simulink model "DIODE_2"  (Simulink 7.7)
settings: Solver=ode15s  StartTime=0.0  StopTime=0.2  MaxStep=0.001  RelTol=1e-3
libraries: fl_lib x18, elec_lib x14, nesl_utility x1
settings Model: Creator=Korisnik  LastModifiedBy=Korisnik

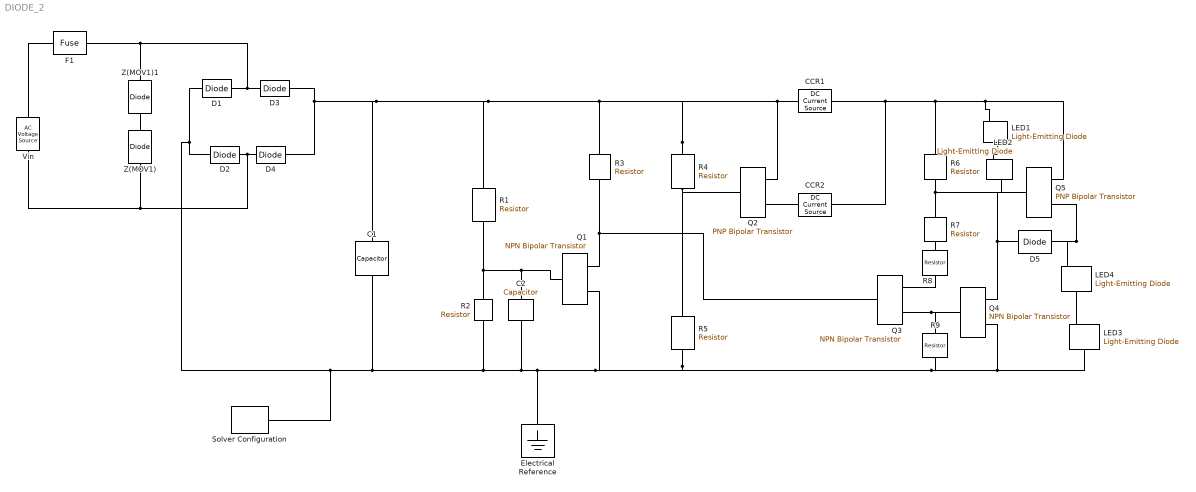
== system DIODE_2 ==
  C1 : fl_lib/Electrical/Electrical Elements/Capacitor  SystemSampleTime=-1  c=2.2 nF  v0=0 V  r=1e-6 Ohm  g=0 1/Ohm  i_Log=off  v_Log=off  vc_Log=off  LocalVarNames=|i|v|vc  LocalVarDescs=|i|v|Internal variable for voltage across capacitor term  LocalVarLogging=[0 0 0]
  C2 : fl_lib/Electrical/Electrical Elements/Capacitor  SystemSampleTime=-1  c=1 nF  v0=0 V  r=1e-6 Ohm  g=0 1/Ohm  i_Log=off  v_Log=off  vc_Log=off  LocalVarNames=|i|v|vc  LocalVarDescs=|i|v|Internal variable for voltage across capacitor term  LocalVarLogging=[0 0 0]
  CCR1 : elec_lib/Additional Components/SPICE-Compatible Components/Sources/DC Current Source  SystemSampleTime=-1  DC=50 mA  current_Log=off  voltage_Log=off  power_Log=off  LocalVarNames=|current|voltage|power  LocalVarDescs=|Current (A)|Voltage (V)|Power (W)  LocalVarLogging=[0 0 0]
  CCR2 : elec_lib/Additional Components/SPICE-Compatible Components/Sources/DC Current Source  SystemSampleTime=-1  DC=30 mA  current_Log=off  voltage_Log=off  power_Log=off  LocalVarNames=|current|voltage|power  LocalVarDescs=|Current (A)|Voltage (V)|Power (W)  LocalVarLogging=[0 0 0]
  D{1..4} (4 alike) : fl_lib/Electrical/Electrical Elements/Diode  SystemSampleTime=-1  Vf=0.68 V  Ron=0.3 Ohm  Goff=1e-8 1/Ohm  i_Log=off  v_Log=off  LocalVarNames=|i|v  LocalVarDescs=|i|v  LocalVarLogging=[0 0]
  D5 : fl_lib/Electrical/Electrical Elements/Diode  SystemSampleTime=-1  Vf=0.6 V  Ron=0.3 Ohm  Goff=1e-8 1/Ohm  i_Log=off  v_Log=off  LocalVarNames=|i|v  LocalVarDescs=|i|v  LocalVarLogging=[0 0]
  Electrical Reference : fl_lib/Electrical/Electrical Elements/Electrical Reference  SystemSampleTime=-1  i_Log=off  LocalVarNames=|i  LocalVarDescs=|i  LocalVarLogging=0
  F1 : elec_lib/Passive Devices/Fuse  SystemSampleTime=-1  I_rated=1 A  T_fuse=0 s  R_closed=0.01 Ohm  G_open=1e-8 1/Ohm  current_Log=off  voltage_Log=off  power_Log=off  LocalVarNames=|current|voltage|power  LocalVarDescs=|Current (A)|Voltage (V)|Power (W)  LocalVarLogging=[0 0 0]
  LED{1..4} (4 alike) : elec_lib/Sensors/Light-Emitting Diode  SystemSampleTime=-1  Gain=0.005 W/A  prmExp=1  I12=[ 0.0017 0.003 ] A  V12=[ 0.9 1.05 ] V  RS=0.1 Ohm  IS=5e-5 A  Tmeas=25 C  ec=10  C_param=1  CJ0=20 pF  VJ=1 V  Mgrad=0.5  Vvec=[ 0.1 10 100 ] V  Cvec=[ 15 10 2 ] pF  FC=0.5  T_param=1  IS_T2=1.8e-4 A  I1_T2=0.0034 A  V1_T2=1.05 V  Tmeas2=125 C  EG_param=1  EG=1.11 eV  XTI_param=1  XTI=3  Tdevice=25 C  LocalVarLogging=[]
  Q1 : elec_lib/Semiconductor Devices/NPN Bipolar Transistor  SystemSampleTime=-1  parameterization=1  prmDatasheet=1  prmEquCoeff=1  BF=100  IS=1e-14 A  VAF=200 V  hfe=100  hoe=5e-5 1/Ohm  Ic_h=1 mA  Vce_h=5 V  V1=0.55 V  I1=0.5 mA  BR=1  Tmeas=25 C  RC=0.01 Ohm  RE=1e-4 Ohm  RB=1 Ohm  C_BC=5 pF  C_BE=5 pF  TF=0 us  TR=0 us  hfe_T2=125  XTB=0  V1_T2=0.45 V  I1_T2=0.5 mA  Tmeas2=125 C  EG=1.11 eV  XTI=3  TdeviceDatasheet=25 C  TdeviceEquCoeff=25 C  LocalVarLogging=[]
  Q2 : elec_lib/Semiconductor Devices/PNP Bipolar Transistor  SystemSampleTime=-1  parameterization=1  prmDatasheet=1  prmEquCoeff=1  BF=100  IS=1e-14 A  VAF=200 V  hfe=100  hoe=5e-5 1/Ohm  Ic_h=-1 mA  Vce_h=-5 V  V1=-0.55 V  I1=-0.5 mA  BR=1  Tmeas=25 C  RC=0.01 Ohm  RE=1e-4 Ohm  RB=1 Ohm  C_BC=5 pF  C_BE=5 pF  TF=0 us  TR=0 us  hfe_T2=125  XTB=0  V1_T2=-0.45 V  I1_T2=-0.5 mA  Tmeas2=125 C  EG=1.11 eV  XTI=3  TdeviceDatasheet=25 C  TdeviceEquCoeff=25 C  LocalVarLogging=[]
  Q3 : elec_lib/Semiconductor Devices/NPN Bipolar Transistor  SystemSampleTime=-1  parameterization=1  prmDatasheet=1  prmEquCoeff=1  BF=100  IS=1e-14 A  VAF=200 V  hfe=100  hoe=5e-5 1/Ohm  Ic_h=1 mA  Vce_h=5 V  V1=0.55 V  I1=0.5 mA  BR=1  Tmeas=25 C  RC=0.01 Ohm  RE=1e-4 Ohm  RB=1 Ohm  C_BC=5 pF  C_BE=5 pF  TF=0 us  TR=0 us  hfe_T2=125  XTB=0  V1_T2=0.45 V  I1_T2=0.5 mA  Tmeas2=125 C  EG=1.11 eV  XTI=3  TdeviceDatasheet=25 C  TdeviceEquCoeff=25 C  LocalVarLogging=[]
  Q4 : elec_lib/Semiconductor Devices/NPN Bipolar Transistor  SystemSampleTime=-1  parameterization=1  prmDatasheet=1  prmEquCoeff=1  BF=100  IS=1e-14 A  VAF=200 V  hfe=100  hoe=5e-5 1/Ohm  Ic_h=1 mA  Vce_h=5 V  V1=0.55 V  I1=0.5 mA  BR=1  Tmeas=25 C  RC=0.01 Ohm  RE=1e-4 Ohm  RB=1 Ohm  C_BC=5 pF  C_BE=5 pF  TF=0 us  TR=0 us  hfe_T2=125  XTB=0  V1_T2=0.45 V  I1_T2=0.5 mA  Tmeas2=125 C  EG=1.11 eV  XTI=3  TdeviceDatasheet=25 C  TdeviceEquCoeff=25 C  LocalVarLogging=[]
  Q5 : elec_lib/Semiconductor Devices/PNP Bipolar Transistor  SystemSampleTime=-1  parameterization=1  prmDatasheet=1  prmEquCoeff=1  BF=100  IS=1e-14 A  VAF=200 V  hfe=100  hoe=5e-5 1/Ohm  Ic_h=-1 mA  Vce_h=-5 V  V1=-0.55 V  I1=-0.5 mA  BR=1  Tmeas=25 C  RC=0.01 Ohm  RE=1e-4 Ohm  RB=1 Ohm  C_BC=5 pF  C_BE=5 pF  TF=0 us  TR=0 us  hfe_T2=125  XTB=0  V1_T2=-0.45 V  I1_T2=-0.5 mA  Tmeas2=125 C  EG=1.11 eV  XTI=3  TdeviceDatasheet=25 C  TdeviceEquCoeff=25 C  LocalVarLogging=[]
  R1 : fl_lib/Electrical/Electrical Elements/Resistor  SystemSampleTime=-1  R=1 MOhm  i_Log=off  v_Log=off  LocalVarNames=|i|v  LocalVarDescs=|i|v  LocalVarLogging=[0 0]
  R2 : fl_lib/Electrical/Electrical Elements/Resistor  SystemSampleTime=-1  R=5.6 kOhm  i_Log=off  v_Log=off  LocalVarNames=|i|v  LocalVarDescs=|i|v  LocalVarLogging=[0 0]
  R3 : fl_lib/Electrical/Electrical Elements/Resistor  SystemSampleTime=-1  R=301 kOhm  i_Log=off  v_Log=off  LocalVarNames=|i|v  LocalVarDescs=|i|v  LocalVarLogging=[0 0]
  R4 : fl_lib/Electrical/Electrical Elements/Resistor  SystemSampleTime=-1  R=590 Ohm  i_Log=off  v_Log=off  LocalVarNames=|i|v  LocalVarDescs=|i|v  LocalVarLogging=[0 0]
  R5 : fl_lib/Electrical/Electrical Elements/Resistor  SystemSampleTime=-1  R=100 kOhm  i_Log=off  v_Log=off  LocalVarNames=|i|v  LocalVarDescs=|i|v  LocalVarLogging=[0 0]
  R6 : fl_lib/Electrical/Electrical Elements/Resistor  SystemSampleTime=-1  R=2.2 kOhm  i_Log=off  v_Log=off  LocalVarNames=|i|v  LocalVarDescs=|i|v  LocalVarLogging=[0 0]
  R7 : fl_lib/Electrical/Electrical Elements/Resistor  SystemSampleTime=-1  R=27 kOhm  i_Log=off  v_Log=off  LocalVarNames=|i|v  LocalVarDescs=|i|v  LocalVarLogging=[0 0]
  R8 : fl_lib/Electrical/Electrical Elements/Resistor  SystemSampleTime=-1  R=27 kOhm  i_Log=off  v_Log=off  LocalVarNames=|i|v  LocalVarDescs=|i|v  LocalVarLogging=[0 0]
  R9 : fl_lib/Electrical/Electrical Elements/Resistor  SystemSampleTime=-1  R=2.2 kOhm  i_Log=off  v_Log=off  LocalVarNames=|i|v  LocalVarDescs=|i|v  LocalVarLogging=[0 0]
  Solver Configuration : nesl_utility/Solver Configuration  SystemSampleTime=-1  PhysicalDomain=network_engine_domain  LeftPortType=input  RightPortType=generic  SubClassName=solver  Accelerate=off  Profile=off  ResidualTolerance=1e-9  MaxNonlinIter=3  MaxModeIter=2  DoFixedCost=off  UseLocalSampling=off  DoDC=off  LinearAlgebra=Sparse  LocalSolverSampleTime=.001  LocalSolverChoice=NE_BACKWARD_EULER_ADVANCER  UseLocalSolver=off
  Vin : fl_lib/Electrical/Electrical Sources/AC Voltage Source  SystemSampleTime=-1  amp=169.71 V  shift=0 rad  omega=60 Hz  i_Log=off  v_Log=off  LocalVarNames=|i|v  LocalVarDescs=|i|v  LocalVarLogging=[0 0]
  Z(MOV1) : elec_lib/Semiconductor Devices/Diode  SystemSampleTime=-1  ModelType=2  Vf=0.6 V  Ron=0.3 Ohm  Goff=1e-8 S  Rz=0.3 Ohm  Vz=150 V  C_PWL=5 pF  prmExp=1  I12=[ 0.0137 0.545 ] A  V12=[ 0.6 0.7 ] V  I1=0.0137 A  V1=0.6 V  RS=0.01 Ohm  IS=1e-12 A  Tmeas=25 C  ec=1  BV=Inf V  C_param=1  CJ0=5 pF  VJ=1 V  Mgrad=0.5  Vvec=[ 0.1 10 100 ] V  Cvec=[ 3.5 1 0.4 ] pF  FC=0.5  T_param=1  IS_T2=1.25e-7 A  I1_T2=0.245 A  V1_T2=0.5 V  Tmeas2=125 C  EG_param=1  EG=1.11 eV  XTI_param=1  XTI=3  dBVdT=0 V/K  Tdevice=25 C  LocalVarLogging=[]
  Z(MOV1)1 : elec_lib/Semiconductor Devices/Diode  SystemSampleTime=-1  ModelType=2  Vf=0.6 V  Ron=0.3 Ohm  Goff=1e-8 S  Rz=0.3 Ohm  Vz=150 V  C_PWL=5 pF  prmExp=1  I12=[ 0.0137 0.545 ] A  V12=[ 0.6 0.7 ] V  I1=0.0137 A  V1=0.6 V  RS=0.01 Ohm  IS=1e-12 A  Tmeas=25 C  ec=1  BV=Inf V  C_param=1  CJ0=5 pF  VJ=1 V  Mgrad=0.5  Vvec=[ 0.1 10 100 ] V  Cvec=[ 3.5 1 0.4 ] pF  FC=0.5  T_param=1  IS_T2=1.25e-7 A  I1_T2=0.245 A  V1_T2=0.5 V  Tmeas2=125 C  EG_param=1  EG=1.11 eV  XTI_param=1  XTI=3  dBVdT=0 V/K  Tdevice=25 C  LocalVarLogging=[]
  connections:
  Vin/RConn1 -- D2/RConn1 -- D4/LConn1 -- Z(MOV1)/LConn1
  F1/LConn1 -- Vin/LConn1
  R9/RConn1 -- Q4/RConn2 -- LED3/RConn1 -- R5/RConn1 -- Q1/RConn2 -- C2/RConn1 -- R2/RConn1 -- C1/RConn1 -- D1/LConn1 -- D2/LConn1 -- Solver Configuration/RConn1 -- Electrical Reference/LConn1
  R3/RConn1 -- Q1/RConn1 -- Q3/LConn1
  R4/RConn1 -- R5/LConn1 -- Q2/LConn1
  CCR2/LConn1 -- Q2/RConn2
  LED1/LConn2 -- R6/LConn1 -- CCR1/RConn1 -- CCR2/RConn1 -- Q5/RConn1
  R6/RConn1 -- R7/LConn1 -- Q5/LConn1
  R7/RConn1 -- R8/LConn1
  R9/LConn1 -- Q3/RConn2 -- Q4/LConn1
  R1/RConn1 -- R2/LConn1 -- C2/LConn1 -- Q1/LConn1
  LED1/RConn1 -- LED2/LConn2
  LED2/RConn1 -- Q4/RConn1 -- D5/LConn1
  R8/RConn1 -- Q3/RConn1
  Q5/RConn2 -- D5/RConn1 -- LED4/LConn2
  CCR1/LConn1 -- D4/RConn1 -- D3/RConn1 -- C1/LConn1 -- R1/LConn1 -- R3/LConn1 -- R4/LConn1 -- Q2/RConn1
  D1/RConn1 -- D3/LConn1 -- F1/RConn1 -- Z(MOV1)1/LConn1
  LED4/RConn1 -- LED3/LConn2
  Z(MOV1)1/RConn1 -- Z(MOV1)/RConn1
